simulink model "NonLinearModel"  (R2023b)
settings: Solver=ode45  StartTime=0.0  StopTime=Tsim*1.4  RelTol=1e-10  EnableMultiTasking=on
values from neighbouring files (symbols this model uses):
  alpha_init = 1*x_trim(1)    [FLYmodel.m]
  b = 9.17    [MyAircraft.mat]    (also in longMotion.m = 2.15; trimConfig.m)
  c = 2.15    [MyAircraft.mat]    (also in trimConfig.m)
  CG = 0.245    [MyAircraft.mat]    (also in trimConfig.m)
  el_init = x_trim(2)    [FLYmodel.m]
  eng_init = x_trim(4)    [FLYmodel.m]
  H_init = plane.h    [FLYmodel.m]
  Jgross = [5000 34000 45000 2200]    [MyAircraft.mat]    (also in trimConfig.m = [Ixx Iyy Izz Ixz])
  longK = lqr(podelny_system,Q,R)    [LQnavrh.m]
  m = 6500    [MyAircraft.mat]    (also in input_param.m = str2double(answerX{3}); trimConfig.m = plane.m)
  pitch_init = 1*x_trim(3)    [FLYmodel.m]
  plane = input_param    [FLYmodel.m]    (also in MyAircraft.mat = )
  rAC = 0.245    [MyAircraft.mat]    (also in trimConfig.m = plane.x_T)
  rho = 0.320310691736    [MyAircraft.mat]    (also in input_param.m = rho_0*(1-vyska/44308)^4.2553; trimConfig.m = plane.rho)
  S = 18.8    [MyAircraft.mat]    (also in latMotion.m; longMotion.m; trimConfig.m)
  Ts = 1/50    (= 0.02)    [FLYmodel.m]
  v0 = plane.v0    [FLYmodel.m]    (also in MyAircraft.mat = 187; input_param.m = str2double(answerX{1}); trimConfig.m)
  V_init = [plane.v0*cos(x_trim(1)) 0 plane.v0*sin(x_trim(1))]'    [FLYmodel.m]
  x_trim = trimConfig(plane)    [FLYmodel.m]    (also in MyAircraft.mat = [0.106204510792 -0.023384072427 0.106204510792 11783.3986038; trimConfig.m = [x(1) x(2) x(3) x(4)])
undefined symbols (not defined in the file or in its folder): Ap, As, Bp, Bs, Cp, Cs, Dp, Ds
libraries: simulink_extras x18
(part 2 of 2)

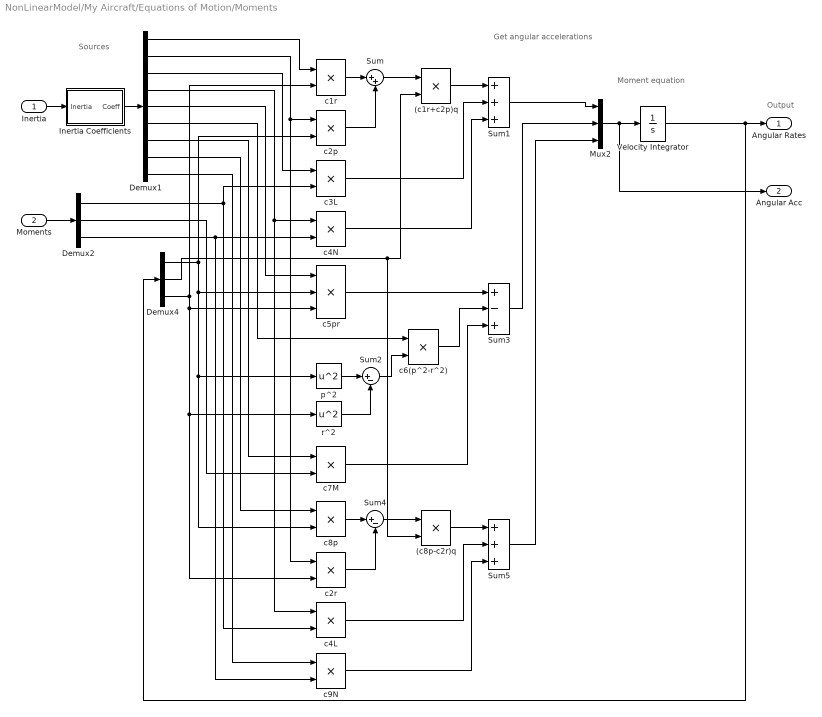
== system NonLinearModel/My Aircraft/Equations of Motion/Moments ==
  note: Sources
  note: Get angular accelerations
  note: Moment equation
  note: Output
  Inertia : Inport  PortDimensions=[4 1]
  Moments : Inport  Port=2  PortDimensions=[3 1]
  (c1r+c2p)q : Product  InputSameDT=on  SaturateOnIntegerOverflow=on  OutDataTypeStr=Inherit: Same as first input
  (c8p-c2r)q : Product  InputSameDT=on  SaturateOnIntegerOverflow=on  OutDataTypeStr=Inherit: Same as first input
  Demux1 : Demux  Outputs=9
      settings: DisplayOption=none
  Demux2 : Demux  Outputs=3
      settings: DisplayOption=none
  Demux4 : Demux  Outputs=3
      settings: DisplayOption=none
  Inertia Coefficients : Subsystem
  Mux2 : Mux  Inputs=3
  Sum : Sum  Inputs=|++  InputSameDT=on  SaturateOnIntegerOverflow=on  OutDataTypeStr=Inherit: Same as first input
  Sum1 : Sum  Inputs=+++  InputSameDT=on  SaturateOnIntegerOverflow=on  OutDataTypeStr=Inherit: Same as first input
  Sum2 : Sum  Inputs=|+-  InputSameDT=on  SaturateOnIntegerOverflow=on  OutDataTypeStr=Inherit: Same as first input
  Sum3 : Sum  Inputs=+-+  InputSameDT=on  SaturateOnIntegerOverflow=on  OutDataTypeStr=Inherit: Same as first input
  Sum4 : Sum  Inputs=|+-  InputSameDT=on  SaturateOnIntegerOverflow=on  OutDataTypeStr=Inherit: Same as first input
  Sum5 : Sum  Inputs=+++  InputSameDT=on  SaturateOnIntegerOverflow=on  OutDataTypeStr=Inherit: Same as first input
  Velocity Integrator : Integrator  InitialCondition=RatesIni
  c1r : Product  InputSameDT=on  SaturateOnIntegerOverflow=on  OutDataTypeStr=Inherit: Same as first input
  c2p : Product  InputSameDT=on  SaturateOnIntegerOverflow=on  OutDataTypeStr=Inherit: Same as first input
  c2r : Product  InputSameDT=on  SaturateOnIntegerOverflow=on  OutDataTypeStr=Inherit: Same as first input
  c3L : Product  InputSameDT=on  SaturateOnIntegerOverflow=on  OutDataTypeStr=Inherit: Same as first input
  c4L : Product  InputSameDT=on  SaturateOnIntegerOverflow=on  OutDataTypeStr=Inherit: Same as first input
  c4N : Product  InputSameDT=on  SaturateOnIntegerOverflow=on  OutDataTypeStr=Inherit: Same as first input
  c5pr : Product  Inputs=3  InputSameDT=on  SaturateOnIntegerOverflow=on  OutDataTypeStr=Inherit: Same as first input
  c6(p^2-r^2) : Product  InputSameDT=on  SaturateOnIntegerOverflow=on  OutDataTypeStr=Inherit: Same as first input
  c7M : Product  InputSameDT=on  SaturateOnIntegerOverflow=on  OutDataTypeStr=Inherit: Same as first input
  c8p : Product  InputSameDT=on  SaturateOnIntegerOverflow=on  OutDataTypeStr=Inherit: Same as first input
  c9N : Product  InputSameDT=on  SaturateOnIntegerOverflow=on  OutDataTypeStr=Inherit: Same as first input
  p^2 : Math  Operator=square  SignedPower=on
  r^2 : Math  Operator=square  SignedPower=on
  Angular Rates : Outport
  Angular Acc : Outport  Port=2
  wires:
  Inertia/1 -> Inertia Coefficients/1(Inertia)
  Inertia Coefficients/1(Coeff) -> Demux1/1
  Demux2/1 -> c4L/2, c3L/2
  Demux2/3 -> c4N/2, c9N/2
  Demux2/2 -> c7M/2
  Moments/1 -> Demux2/1
  Demux1/1 -> c1r/1
  c1r/1 -> Sum/1
  c2p/1 -> Sum/2
  Sum/1 -> (c1r+c2p)q/1
  (c1r+c2p)q/1 -> Sum1/1
  c3L/1 -> Sum1/2
  c4N/1 -> Sum1/3
  Sum1/1 -> Mux2/1
  Demux1/5 -> c5pr/1
  p^2/1 -> Sum2/1
  r^2/1 -> Sum2/2
  Demux1/6 -> c6(p^2-r^2)/1
  Sum2/1 -> c6(p^2-r^2)/2
  Demux1/7 -> c7M/1
  c5pr/1 -> Sum3/1
  c6(p^2-r^2)/1 -> Sum3/2
  c7M/1 -> Sum3/3
  Demux1/8 -> c8p/1
  Demux4/1 -> c2p/2, c5pr/2, c8p/2, p^2/1
  c8p/1 -> Sum4/1
  c2r/1 -> Sum4/2
  Sum4/1 -> (c8p-c2r)q/1
  Demux1/4 -> c4N/1, c4L/1
  Demux1/9 -> c9N/1
  (c8p-c2r)q/1 -> Sum5/1
  c4L/1 -> Sum5/2
  c9N/1 -> Sum5/3
  Sum5/1 -> Mux2/3
  Mux2/1 -> Angular Acc/1, Velocity Integrator/1
  Demux1/2 -> c2p/1, c2r/1
  Demux1/3 -> c3L/1
  Demux4/3 -> c1r/2, c2r/2, r^2/1, c5pr/3
  Demux4/2 -> (c1r+c2p)q/2, (c8p-c2r)q/2
  Sum3/1 -> Mux2/2
  Velocity Integrator/1 -> Angular Rates/1, Demux4/1

== system NonLinearModel/My Aircraft/Sum forces and moments/Total Acceleration ==
  note: Sources
  Faero : Inport  PortDimensions=[3 1]
  Mass : Inport  Port=2  PortDimensions=1
  Engine : Inport  Port=3
  F/m : Product  Inputs=*/  InputSameDT=on  SaturateOnIntegerOverflow=on  OutDataTypeStr=Inherit: Same as first input
  Ground : Ground
  Mux : Mux  Inputs=3
  Sum : Sum  Inputs=|++
  Acc : Outport
  wires:
  Faero/1 -> Sum/1
  Mass/1 -> F/m/2
  F/m/1 -> Acc/1
  Sum/1 -> F/m/1
  Engine/1 -> Mux/1
  Mux/1 -> Sum/2
  Ground/1 -> Mux/2, Mux/3

== system NonLinearModel/My Aircraft/Sum forces and moments/Total Moment ==
  note: Moments at CG created by aero and propulsion forces
  note: Sources
  Faero : Inport  PortDimensions=[3 1]
  Maero : Inport  Port=2  PortDimensions=[3 1]
  CGpos : Inport  Port=3
  Demux : Demux  Outputs=[1 1 1]
      settings: DisplayOption=none
  Mux2 : Mux  Inputs=3
  Product : Product  InputSameDT=on  SaturateOnIntegerOverflow=on  OutDataTypeStr=Inherit: Same as first input
  Selector : Selector  InputPortWidth=3  IndexOptions=Index vector (dialog)  Indices=3  OutputSizes=[(-2)]
  Sum1 : Sum  Inputs=2  InputSameDT=on  SaturateOnIntegerOverflow=on  OutDataTypeStr=Inherit: Same as first input
  Sum2 : Sum  Inputs=|+-  InputSameDT=on  SaturateOnIntegerOverflow=on  OutDataTypeStr=Inherit: Same as first input
  phugoid : Gain  Gain=-c
  r_aero : Constant  Value=rAC
  Mcg : Outport
  wires:
  CGpos/1 -> Sum2/2
  r_aero/1 -> Sum2/1
  Faero/1 -> Selector/1
  Mux2/1 -> Mcg/1
  Maero/1 -> Demux/1
  Demux/2 -> Sum1/2
  Selector/1 -> phugoid/1
  Sum2/1 -> Product/2
  Product/1 -> Sum1/1
  Demux/1 -> Mux2/1
  Sum1/1 -> Mux2/2
  Demux/3 -> Mux2/3
  phugoid/1 -> Product/1

== system NonLinearModel/Controls/Subsystem/PAH_LQ/Subsystem ==
  velocity : Inport
  states : Inport  Port=2
  altitude : Inport  Port=3
  2-D Lookup Table{,1..3} (4 alike) : Lookup_n-D  BreakpointsForDimension1=[1:3]  BreakpointsForDimension2=[1:3]  InternalRulePriority=Speed  RndMeth=Simplest
      settings: InputPortMap=u0,u1
  MATLAB Function : MATLAB Function  TreatAsAtomicUnit=on
  Mux : Mux
  y : Outport
  wires:
  altitude/1 -> 2-D Lookup Table3/2, 2-D Lookup Table2/2, 2-D Lookup Table1/2, 2-D Lookup Table/2
  velocity/1 -> 2-D Lookup Table3/1, 2-D Lookup Table2/1, 2-D Lookup Table1/1, 2-D Lookup Table/1
  states/1 -> MATLAB Function/2(states)
  2-D Lookup Table/1 -> Mux/1
  2-D Lookup Table1/1 -> Mux/2
  2-D Lookup Table2/1 -> Mux/3
  2-D Lookup Table3/1 -> Mux/4
  Mux/1 -> MATLAB Function/1(gains)  "scheduled gains"
  MATLAB Function/1(y) -> y/1

== system NonLinearModel/Controls/Subsystem/demuxing hell/Zero Offset ==
  In : Inport
  Abs : Abs
  Constant : Constant  Value=tol
  Non-zero Sign : Subsystem  mask(Non-zero sign){}
      mask help: Sign function outputs 1 for input greater than or equal to 0, and -1 otherwise.
  Product : Product  InputSameDT=on  SaturateOnIntegerOverflow=on  OutDataTypeStr=Inherit: Same as first input
  Switch : Switch  Threshold=tol
  Out : Outport
  wires:
  Switch/1 -> Out/1
  Product/1 -> Switch/3
  Constant/1 -> Product/2
  Non-zero Sign/1(Out) -> Product/1
  Abs/1 -> Switch/2
  In/1 -> Abs/1, Non-zero Sign/1(In), Switch/1

== system NonLinearModel/My Aircraft/Aerodynamic model/Wind-axes Velocities/Vector norm ==
  Vec : Inport
  Dot Product : DotProduct  OutDataTypeStr=Inherit: Inherit via internal rule
  Math Function : Math  Operator=sqrt  SignedPower=on
  Mag : Outport
  wires:
  Dot Product/1 -> Math Function/1
  Vec/1 -> Dot Product/1, Dot Product/2
  Math Function/1 -> Mag/1

== system NonLinearModel/My Aircraft/Aerodynamic model/Wind-axes Velocities/Zero Offset ==
  In : Inport
  Abs : Abs
  Constant : Constant  Value=tol
  Non-zero Sign : Subsystem  mask(Non-zero sign){}
      mask help: Sign function outputs 1 for input greater than or equal to 0, and -1 otherwise.
  Product : Product  InputSameDT=on  SaturateOnIntegerOverflow=on  OutDataTypeStr=Inherit: Same as first input
  Switch : Switch  Threshold=tol
  Out : Outport
  wires:
  Switch/1 -> Out/1
  Product/1 -> Switch/3
  Constant/1 -> Product/2
  Non-zero Sign/1(Out) -> Product/1
  Abs/1 -> Switch/2
  In/1 -> Abs/1, Non-zero Sign/1(In), Switch/1

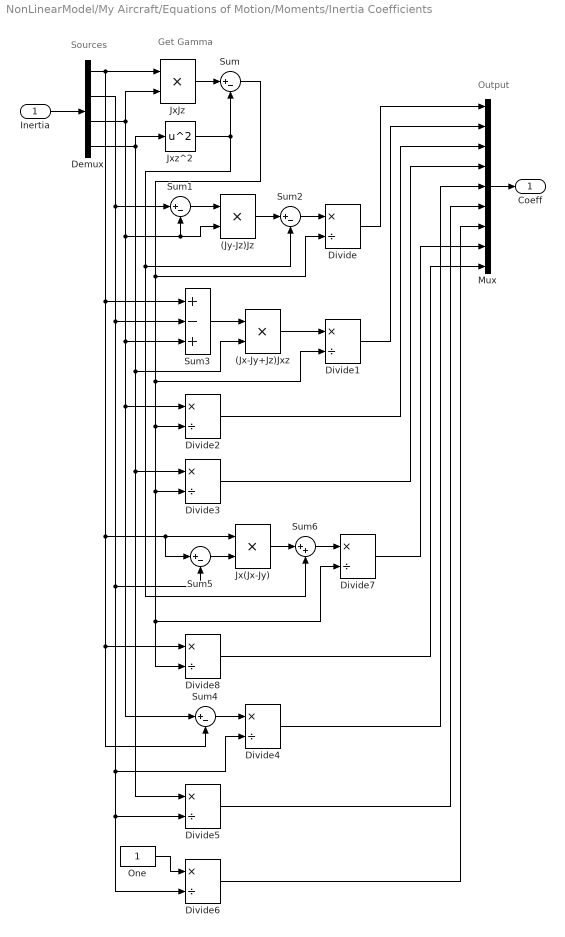
== system NonLinearModel/My Aircraft/Equations of Motion/Moments/Inertia Coefficients ==
  note: Sources
  note: Get Gamma
  note: Output
  Inertia : Inport  PortDimensions=[4 1]
  (Jx-Jy+Jz)Jxz : Product  InputSameDT=on  SaturateOnIntegerOverflow=on  OutDataTypeStr=Inherit: Same as first input
  (Jy-Jz)Jz : Product  InputSameDT=on  SaturateOnIntegerOverflow=on  OutDataTypeStr=Inherit: Same as first input
  Demux : Demux
      settings: DisplayOption=none
  Divide{,1..8} (9 alike) : Product  Inputs=*/  InputSameDT=on  SaturateOnIntegerOverflow=on  OutDataTypeStr=Inherit: Same as first input
  Jx(Jx-Jy) : Product  InputSameDT=on  SaturateOnIntegerOverflow=on  OutDataTypeStr=Inherit: Same as first input
  JxJz : Product  InputSameDT=on  SaturateOnIntegerOverflow=on  OutDataTypeStr=Inherit: Same as first input
  Jxz^2 : Math  Operator=square  SignedPower=on
  Mux : Mux  Inputs=9
  One : Constant
  Sum{,1..2,4..5} (5 alike) : Sum  Inputs=|+-  InputSameDT=on  SaturateOnIntegerOverflow=on  OutDataTypeStr=Inherit: Same as first input
  Sum3 : Sum  Inputs=+-+  InputSameDT=on  SaturateOnIntegerOverflow=on  OutDataTypeStr=Inherit: Same as first input
  Sum6 : Sum  Inputs=|++  InputSameDT=on  SaturateOnIntegerOverflow=on  OutDataTypeStr=Inherit: Same as first input
  Coeff : Outport
  wires:
  Demux/3 -> Sum4/1, Divide2/1, Sum3/3, Sum1/2, (Jy-Jz)Jz/2, JxJz/2
  Inertia/1 -> Demux/1
  Demux/1 -> Sum5/1, Jx(Jx-Jy)/1, Sum4/2, Divide8/1, Sum3/1, JxJz/1
  Demux/2 -> Sum5/2, Divide6/2, Divide5/2, Divide4/2, Sum3/2, Sum1/1
  Demux/4 -> Divide5/1, Divide3/1, (Jx-Jy+Jz)Jxz/2, Jxz^2/1
  JxJz/1 -> Sum/1
  Jxz^2/1 -> Sum6/2, Sum2/2, Sum/2
  Sum/1 -> Divide8/2, Divide7/2, Divide3/2, Divide2/2, Divide1/2, Divide/2
  Sum1/1 -> (Jy-Jz)Jz/1
  (Jy-Jz)Jz/1 -> Sum2/1
  Sum2/1 -> Divide/1
  Divide/1 -> Mux/1
  Sum3/1 -> (Jx-Jy+Jz)Jxz/1
  (Jx-Jy+Jz)Jxz/1 -> Divide1/1
  Divide1/1 -> Mux/2
  Divide2/1 -> Mux/3
  Divide3/1 -> Mux/4
  Sum4/1 -> Divide4/1
  Divide4/1 -> Mux/5
  Divide5/1 -> Mux/6
  One/1 -> Divide6/1
  Divide6/1 -> Mux/7
  Jx(Jx-Jy)/1 -> Sum6/1
  Sum6/1 -> Divide7/1
  Divide7/1 -> Mux/8
  Sum5/1 -> Jx(Jx-Jy)/2
  Divide8/1 -> Mux/9
  Mux/1 -> Coeff/1

== system NonLinearModel/Controls/Subsystem/demuxing hell/Zero Offset/Non-zero Sign ==
  In : Inport
  One : Constant
  Relational Operator : RelationalOperator  Operator===
  Sign : Signum
  Switch : Switch  Threshold=1
  Zero : Constant  Value=0
  Out : Outport
  wires:
  Switch/1 -> Out/1
  Sign/1 -> Switch/3
  One/1 -> Switch/1
  Relational Operator/1 -> Switch/2
  In/1 -> Sign/1, Relational Operator/1
  Zero/1 -> Relational Operator/2

== system NonLinearModel/My Aircraft/Aerodynamic model/Wind-axes Velocities/Zero Offset/Non-zero Sign ==
  In : Inport
  One : Constant
  Relational Operator : RelationalOperator  Operator===
  Sign : Signum
  Switch : Switch  Threshold=1
  Zero : Constant  Value=0
  Out : Outport
  wires:
  Switch/1 -> Out/1
  Sign/1 -> Switch/3
  One/1 -> Switch/1
  Relational Operator/1 -> Switch/2
  In/1 -> Sign/1, Relational Operator/1
  Zero/1 -> Relational Operator/2

== matlab function NonLinearModel/Controls/Subsystem/PAH_LQ/Subsystem/MATLAB Function ==
  data: gains input; y output; states input
function y = fcn(gains, states)

y  = gains*states';

== matlab function NonLinearModel/My Aircraft/Aerodynamic model/Embedded MATLAB Function ==
  data: Wind input; CX output; Control input; ABdot input; AngRates input; Mach input; mass input; CY output; CZ output; Cl output; Cm output; Cn output; rho input; M_const input
function [CX,CY,CZ,Cl,Cm,Cn] = AeroCoefM(Wind,Control,ABdot,AngRates,Mach,mass,rho,M_const)

V = Wind(1);
beta = Wind(2);
alpha = Wind(3);
de = Control(1);
da = Control(2);
dr = Control(3);
M = Mach;
m = mass;
c = 2.15; % m
S = 18.8; 
b = 9.17;

p = AngRates(1);
q = AngRates(2);
r = AngRates(3);
adot = ABdot(1);
m = mass; 

%% Drag
% Minimum drag
if M<0.4
    CD0 = 0.0223;
elseif M>0.92 
    CD0 = 0.1032;
else
    CD0 = 7.861*M^4 - 18.378*M^3 + 15.832*M^2 - 5.9269*M + 0.8349;
%     CD0 = 7.861*M_const^4 - 18.378*M_const^3 + 15.832*M_const^2 ...
%         - 5.9269*M_const + 0.8349;
end

% alpha derivate
    CDa = 0.00103*(alpha*180/pi)^2 - 0.00308*alpha*180/pi;


% Pitch control (elevator) derivative
CDde = 6.2863E-07*(de*180/pi)^3 + 4.1831E-05*(de*180/pi)^2 -...
    3.1917E-04*(de*180/pi) + 1.6834E-04;


%% Lift
% Zero-alpha lift
    % CL0 = 0.3;
    x_cy0       = [0,0.4,0.6,0.7,0.75,0.8,0.85,0.9]; 
    y_cy0       = [0.09,0.09,0.09,0.105,0.13,0.12,0.07,0.02];
    % pocatecni hodnota vztlakoveho soucinitele
%     CL0 = interp1(x_cy0,y_cy0,M_const);
    CL0 = interp1(x_cy0,y_cy0,M);
    
% alpha derivative
    % CLa = 4.44;
    % derivace soucinitele vztlaku podle uhlu nabehu
    if M <= 0.3
        CLa = 4.4418;
    else
        CLa = - 62.716*M^5 + 122.09*M^4 - 85.797*M^3 + 28.153*M^2 ...
                   - 3.8433*M + 4.541;
    end
% Pitch control (elevator) derivative
    CLde = 0.305;

% alpha-dot derivative
    % CLalphadot = 0;
    % derivace soucinitele vztlaku podle bezrozmerne zmeny uhlu nabehu
    if M<0.3
        Mp = 0.3;
        CLalphadot = -49.167 + 558.542*Mp - 2284.051*Mp^2 ... 
        + 4412.037*Mp^3 - 4067.130*Mp^4 + 1435.185*Mp^5;
    elseif M>0.7
        Mp = 0.7;
        CLalphadot = -49.167 + 558.542*Mp - 2284.051*Mp^2 ... 
        + 4412.037*Mp^3 - 4067.130*Mp^4 + 1435.185*Mp^5;
    else
        CLalphadot = -49.167 + 558.542*M - 2284.051*M^2 ... 
        + 4412.037*M^3 - 4067.130*M^4 + 1435.185*M^5;
    end
% Pitch rate derivative
    % CLq = 3.8;
    % derivace soucinitele vztlaku podle bezrozmerne rychlosti kloneni
%     CLq = 5.7414 - 9.3115*M + 20.8*M^2 - 13.465*M^3;
    tx_M        = [0.0, 0.3, 0.4, 0.5, 0.6, 0.7, 0.75, 0.9];
    tc_y_w      = [4.45, 4.45, 4.5, 4.6, 4.7, 4.85, 4.75, 4.75];
    CLq = interp1(tx_M,tc_y_w,M);


%%% Pitch moment coefficient %%%
% Zero-alpha pitch
    % Cm0 = 0;
    y_mz0 = [0.025,0.025,0.03,0.025,0.02,0.05,-0.02,-0.03];
%     pocatecni hodnota klopiveho soucinitele
%     Cm0 = interp1(x_cy0,y_mz0,M);
    Cm0 = interp1(x_cy0,y_mz0,M_const);
%     Cm0 = 0.025;
% 	if M <= 0.3
%         Cm0 = 0.025;
%     else
%         Cm0 = -0.703*M^3 + 0.828*M^2 - 0.258*M + 0.040;
%     end
    
% alpha derivative
    % Cma = -0.683;
    if M <= 0.3
        Cma = -0.4899;
    else
%         M = M_const;
        Cma = 5.9964*M^4 - 10.271*M^3 + 6.7921*M^2 - 2.0056*M -0.2708;
    end    

% Pitch control derivative
    Cmde = -0.88;
    
% alpha_dot derivative
%     Cmalphadot = -4.36;
    if M <= 0.3
        Cmalphadot = -1.38271969;
    else
        Cmalphadot = 502.427*M^5 - 1303.11*M^4 + 1330.2481*M^3 ...
            - 668.0225*M^2 + 164.08*M - 17.0671;
    end    
% Pitch rate derivative
%     Cmq = -9.96;
    if M <= 0.3
        Cmq = -4.9934668;
    else
        Cmq = 2.5926*M^3 - 8.7063*M^2 + 4.8590*M - 5.7376;
    end    

%% Side force coefficient %%%
    cyPom = m*9.81/(0.5*rho*V^2*S);
    % Sideslip derivative
    % CYbeta = -0.564;
    CYbeta = (-0.946 - 0.0333*cyPom + 0.0032*M - 0.16*M^2);
    % Roll control derivative
    CYda = -0.02;
    % Yaw control derivative
    CYdr = (-0.1845 + 0.0325*cyPom -0.0093*M -0.0228*M^2 ...
        -0.012*M^3);

%% Roll moment coefficient %%%
    % Sideslip derivative
    if M<0.45
        Clbeta = -0.056 - 0.0576*cyPom - 0.0088*M;
    else
        Clbeta = -0.06 - 0.0576*cyPom - 0.0285*(M - 0.45);
    end
    
    % Roll control derivative
    if M<=0.6
        Clda = (-0.156 + 0.04*(M -0.2));
    else
        Clda = -1.1039 + 4.6696*M - 7.5941*M^2 ...
            + 4.1483*M^3;
    end
    
    % Yaw control derivative
    Cldr = (-0.03 + 0.008*cyPom)*1;
    
    % Roll rate derivative
    Clp = -0.5365 - 1.5267*M + 10.781*M^2 ...
        -20.666*M^3 + 12.4242*M^4;
    % Yaw rate derivative
    Clr = (-0.075 - 0.215*cyPom -0.016*M);

%% Yaw moment coefficient %%%
    % Sideslip derivative
    Cnbeta = (-0.173 + 0.01667*cyPom + 0.0092*M -0.1*M^2 +...
        0.0208*M^3);
    
    % Roll control derivative   
    Cnda = -0.0015;
    
    % Yaw control derivative
    Cndr = (0.015*cyPom - 0.095 -0.0056*M -0.0089*M^2 ...
        - 0.0068*M^3);
    
    % Roll rate derivative
    if M<0.7
        Cnp = -0.07435 + 0.045*cyPom - 0.0092*M;
    else
        Cnp = -0.08079 + 0.044*cyPom - 0.0333*(M-0.7);
    end

    % Yaw rate derivative
    Cnr = -0.2291 - 0.0065*cyPom -0.0236*cyPom^2 + 0.0069*cyPom^3 ...
            - 0.0219*M + 0.0097*M^2 - 0.0447*M^3;

CX = CD0 + CDa + CDde;
CY = CYbeta*beta + CYda*da + CYdr*dr;
CZ = CL0 + CLa*alpha + CLde*de + c*q*CLq/V + c*adot*CLalphadot/V;
Cl = Clbeta*beta + b*p*Clp/(2*V) + b*r*Clr/(2*V) + Clda*da + Cldr*dr;
Cm = Cm0 + Cma*alpha + Cmde*de + c*q*Cmq/V + c*adot*Cmalphadot/V;
Cn = Cnbeta*beta + b*p*Cnp/(2*V) + b*r*Cnr/(2*V) + Cnda*da + Cndr*dr;
